simulink model "zad3_3_5"  (Simulink 6.5)
settings: Solver=ode45  StartTime=0.0  StopTime=10.0  RelTol=1e-3
settings Model: Creator=rr44283  LastModifiedBy=rr44283

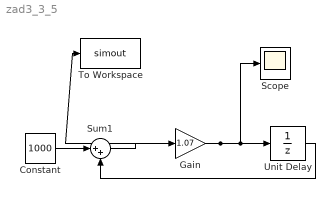
== system zad3_3_5 ==
  Constant : Constant  Value=1000  OutDataType=sfix(16)  ConRadixGroup=Use specified scaling  OutScaling=2^0  SampleTime=inf  FramePeriod=inf
  Gain : Gain  Gain=1.07
  Scope : Scope
  Sum1 : Sum  Inputs=|++
  To Workspace : ToWorkspace  VariableName=simout  SampleTime=-1  SaveFormat=Structure
  Unit Delay : UnitDelay
  wires:
  Sum1/1 -> Gain/1
  Gain/1 -> Unit Delay/1, Scope/1, To Workspace/1
  Unit Delay/1 -> Sum1/2
  Constant/1 -> Sum1/1
